simulink model "testNetworkParseInC"  (R2015b)
settings: Solver=FixedStepDiscrete  StartTime=0.0  StopTime=Inf  FixedStep=0.001  RelTol=1e-3
undefined symbols (not defined in the file or in its folder): gcbh, mxpcnbunlink, mxpcrtudprx
libraries: slrtlib x5, xpciplib x2, libBusSerialize x1, dspindex x1, xpcnetworkbufferlib x1
settings Model: xpc_rtwmakecfg_data=_xpciplib__xpcnblib__xpcetherlib__xpcether8255xlib__xpcetherGbElib_  SimulationMode=external  Creator=djoshea  LastModifiedBy=shenoylab
settings SolverCC: EnableConcurrentExecution=on
settings DataIOCC: SaveFormat=Array
settings OptimizationCC: BlockReduction=off  OptimizeBlockIOStorage=off  BufferReuse=off  GlobalBufferReuse=off  ExpressionFolding=off  LocalBlockOutputs=off  SimCompilerOptimization=on
settings HardwareCC: ProdBitPerPointer=32  ProdLargestAtomicFloat=None  ProdWordSize=32  ProdLongLongMode=on  ProdHWDeviceType=Generic->32-bit x86 compatible  TargetBitPerLong=64  TargetBitPerPointer=64  TargetIntDivRoundTo=Zero  TargetEndianess=LittleEndian  TargetWordSize=64  TargetHWDeviceType=Intel->x86-64
settings SFSimCC: SimBuildMode=sf_nonincremental_build
settings RTWCC: SystemTargetFile=slrt.tlc  TemplateMakefile=slrt_default_tmf  Description=Simulink Real-Time  GenerateReport=on  CustomSource=cerebusParse.c  LaunchReport=on  RTWCompilerOptimization=on
settings CodeAppCC: MaxIdLength=95
settings SimulinkRealTimeCC: GeneratePreprocessorConditionals=Disable all
settings ConfigComp: CovModelRefEnable=Off

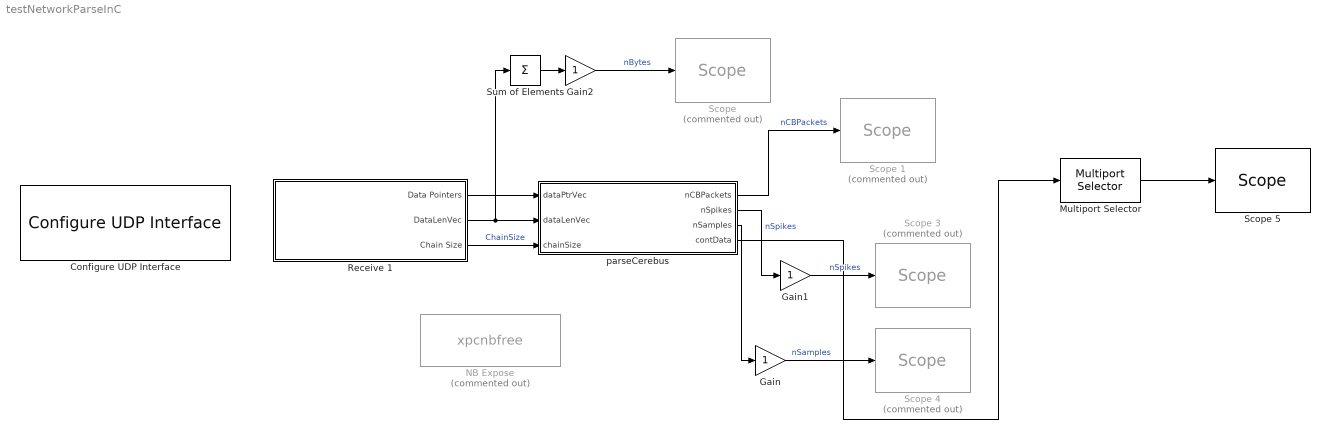
== system testNetworkParseInC ==
  Configure UDP Interface : libBusSerialize/Configure UDP Interface  PoolSizes=[8196 512 4096 65535]  ID=2  udpID=0  IpAddress='192.168.137.4'  SubnetMask=255.255.255.0  Gateway=0.0.0.0  EthDrv=Intel Gigabit  PciBus=4  PciSlot=4
  Gain : Gain  OutDataTypeStr=double
  Gain1 : Gain  OutDataTypeStr=double
  Gain2 : Gain  OutDataTypeStr=double
  Multiport Selector : dspindex/Multiport Selector  rowsOrCols=Columns  idxCellArray={ 1 }  idxErrMode=Clip Index
  NB Expose : S-Function  Commented=on  InitFcn=mxpcnbunlink(1,0);  FunctionName=xpcnbfree  SFunctionDeploymentMode=off  EnableBusSupport=off  mask(xpcnbunlink){}
      mask help: Unlink a chain into a vector of network buffers.
      mask Help: eval('xpcdoc(''NB_Unlink'')');
      mask DialogControl DescGroupVar Prompt: Network Buffer Free
      mask Display: disp('NB Free');
  Receive 1 : Subsystem  InitFcn=mxpcrtudprx(1, get_param(gcbh, 'ID'));  mask(rtudpreceive){ID=1, Receive1=0.0.0.0, Receive2=1002, maxPackets=100, Receive4=0.001, udpID=0}
      mask prompts: ID "Device ID:"; Receive1 "Source IP Address:"; Receive2 "Local (destination) port:"; maxPackets "Max Packets"; Receive4 "Sample time:"; udpID "Internal UDP ID:"
      mask help:
      | Receive data over UDP network on a dedicated network interface.
      |
      | This block receives data on the specified local (destination) port. To receive all data sent to this port, set 'Source IP Address' to 0.0.0.0. To receive data sent to this port from a specific remote source, enter the IP address of that source.
      mask init:
      | Receive1 = ipaddr(Receive1);
      | udpID = ID -1;
      mask Help: eval('xpcdoc(''RT_UDP_RECEIVE'')');
      mask TypeOptions ID: 1 | 2 | 3 | 4 | 5 | 6 | 7 | 8
      mask Display:
      | disp('UDP Expose\nId: 1');
      | port_label('output', 1, 'DataPtrVec');
      | port_label('output', 2, 'DataLenVec');
      | port_label('output', 3, 'Chain Size');
  "Scope " : slrtlib/Displays and Logging/Scope   Commented=on  scopeno=1  scopetype=Target  autostart=on  viewmode=Graphical rolling  formatstr='%15.6f'  grid=on  ylimits=[0 0]  nosamples=1000  noprepostsamples=0  interleave=1  triggermode=FreeRun  triggersignal=1  trigsignalfromport=off  triggerlevel=0.0  triggerslope=Either  triggerscope=1  triggersample=0  filename=data.dat  mode=Lazy  writesize=512  autorestart=off  dynamicfilemode=off  maxwritefilesize=512*1024^2
  Scope 1 : slrtlib/Displays and Logging/Scope   Commented=on  scopeno=2  scopetype=Target  autostart=on  viewmode=Graphical rolling  formatstr='%15.6f'  grid=on  ylimits=[0 100]  nosamples=1000  noprepostsamples=0  interleave=1  triggermode=FreeRun  triggersignal=1  trigsignalfromport=off  triggerlevel=0.0  triggerslope=Either  triggerscope=1  triggersample=0  filename=data.dat  mode=Lazy  writesize=512  autorestart=off  dynamicfilemode=off  maxwritefilesize=512*1024^2
  Scope 3 : slrtlib/Displays and Logging/Scope   Commented=on  scopeno=4  scopetype=Target  autostart=on  viewmode=Graphical rolling  formatstr='%15.6f'  grid=on  ylimits=[0 0]  nosamples=1000  noprepostsamples=0  interleave=1  triggermode=FreeRun  triggersignal=1  trigsignalfromport=off  triggerlevel=0.0  triggerslope=Either  triggerscope=1  triggersample=0  filename=data.dat  mode=Lazy  writesize=512  autorestart=off  dynamicfilemode=off  maxwritefilesize=512*1024^2
  Scope 4 : slrtlib/Displays and Logging/Scope   Commented=on  scopeno=5  scopetype=Target  autostart=on  viewmode=Graphical rolling  formatstr='%15.6f'  grid=on  ylimits=[0 0]  nosamples=1000  noprepostsamples=0  interleave=1  triggermode=FreeRun  triggersignal=1  trigsignalfromport=off  triggerlevel=0.0  triggerslope=Either  triggerscope=1  triggersample=0  filename=data.dat  mode=Lazy  writesize=512  autorestart=off  dynamicfilemode=off  maxwritefilesize=512*1024^2
  Scope 5 : slrtlib/Displays and Logging/Scope   scopeno=6  scopetype=Target  autostart=on  viewmode=Graphical rolling  formatstr='%15.6f'  grid=on  ylimits=[0 0]  nosamples=5000  noprepostsamples=0  interleave=1  triggermode=FreeRun  triggersignal=1  trigsignalfromport=off  triggerlevel=0.0  triggerslope=Either  triggerscope=1  triggersample=0  filename=data.dat  mode=Lazy  writesize=512  autorestart=off  dynamicfilemode=off  maxwritefilesize=512*1024^2
  Sum of Elements : Sum  Inputs=+
  parseCerebus : MATLAB Function  TreatAsAtomicUnit=on
  wires:
  Receive 1/2(DataLenVec) -> parseCerebus/2(dataLenVec), Sum of Elements/1
  Sum of Elements/1 -> Gain2/1
  Receive 1/1(Data Pointers) -> parseCerebus/1(dataPtrVec)
  Receive 1/3(Chain Size) -> parseCerebus/3(chainSize)  "ChainSize"
  parseCerebus/1(nCBPackets) -> Scope 1/1  "nCBPackets"
  parseCerebus/2(nSpikes) -> Gain1/1  "nSpikes"
  parseCerebus/3(nSamples) -> Gain/1
  Gain/1 -> Scope 4/1  "nSamples"
  Gain1/1 -> Scope 3/1  "nSpikes"
  Gain2/1 -> "Scope "/1  "nBytes"
  parseCerebus/4(contData) -> Multiport Selector/1
  Multiport Selector/1 -> Scope 5/1

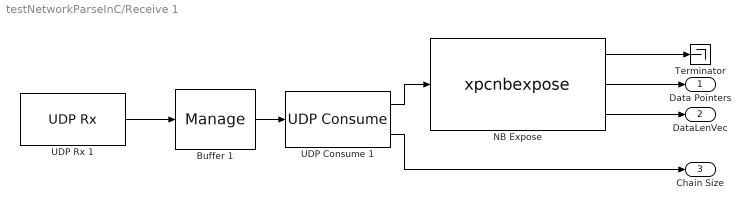
== system testNetworkParseInC/Receive 1 ==
  Buffer 1 : xpcnetworkbufferlib/Manage   ChainSize=maxPackets  BufferSize=maxPackets*5  Threshold=0
  NB Expose : S-Function  InitFcn=mxpcnbunlink(1,0);  FunctionName=xpcnbexpose  Parameters=vectorLength  SFunctionDeploymentMode=off  EnableBusSupport=off  mask(xpcnbunlink){VectorLength=maxPackets}
      mask prompts: VectorLength "Vector length (-1 inherit):"
      mask help: Unlink a chain into a vector of network buffers.
      mask init:
      | [vectorLength] = mxpcnbunlink(2, VectorLength);
      mask Help: eval('xpcdoc(''NB_Unlink'')');
      mask Display:
      | disp('NB Expose');
      | port_label('output', 1, 'NBVec');
      | port_label('output', 2, 'DataPtrVec');
      | port_label('output', 3, 'DataLenVec');
  Terminator : Terminator
  UDP Consume 1 : xpciplib/UDP Consume   Group=udpID  VectorSize=0  SampleTime=Receive4
  UDP Rx 1 : xpciplib/UDP Rx   Priority=5  Group=udpID  sip=Any  SourceAddress=Receive1  lup=Specify  LocalPort=Receive2  SampleTime=Receive4
  Data Pointers : Outport
  DataLenVec : Outport  Port=2
  Chain Size : Outport  Port=3
  wires:
  UDP Consume 1/1 -> NB Expose/1
  Buffer 1/1 -> UDP Consume 1/1
  UDP Rx 1/1 -> Buffer 1/1
  UDP Consume 1/2 -> Chain Size/1
  NB Expose/1 -> Terminator/1
  NB Expose/2 -> Data Pointers/1
  NB Expose/3 -> DataLenVec/1

== matlab function testNetworkParseInC/parseCerebus ==
  data: dataPtrVec input; dataLenVec input; chainSize input; nCBPackets output; nSpikes output; nSamples output; contData output
function [nCBPackets, nSpikes, nSamples, contData] = parseCerebus(dataPtrVec, dataLenVec, chainSize)
%#codegen

% these pointers are coder.opaque, they will be used only via ceval calls
% within CerebusParse
% [pp, pBufferEnd] = CerebusParse.nbExtractPacketData(nb);

maxSpikes = 1000;
spikeData = zeros(48, maxSpikes, 'int16');
nSpikes = uint32(0);

maxContSamples = 30;
maxChannels = 128;
contData = zeros(maxChannels, maxContSamples, 'int16');
nSamples = uint32(0);

% nbVecOut = nbVec;
nCBPackets = uint32(0);

for iP = uint32(1):uint32(chainSize)
    if dataPtrVec(iP) == 0 || dataLenVec(iP) == 0
        continue;
    end
    
    [pp, pBufferEnd] = CerebusParse.getPointersFromDataPtr(dataPtrVec(iP), dataLenVec(iP));
    nCBPackets = nCBPackets + uint32(1);
    
    while true
        if CerebusParse.isSpikePacket(pp)
            if nSpikes < maxSpikes
                nSpikes = nSpikes + uint32(1);
                spikeData = CerebusParse.copySpikeWaveformToBufferColumn(pp, spikeData, nSpikes);
            end

        elseif CerebusParse.isContinuousPacketForGroup(pp, uint8(5))
            if nSamples < maxContSamples
                nSamples = nSamples + uint32(1);
                contData = CerebusParse.copyContinuousSamplesToBufferColumn(pp, contData, nSamples);
%                 contData(:, nSamples) = contData(:, nSamples) - mean(contData([1:32 1:32 1:32 1:32], nSamples));
            end
        end

        if ~CerebusParse.hasNext(pp, pBufferEnd)
            break;
        end
        pp = CerebusParse.getNext(pp);
        nCBPackets = nCBPackets + uint32(1);
    end
end

% contData = samplesP(numSamplesP, :) - mean(samplesP(numSamplesP, :));

% CerebusParse.nbFree(nb);
